simulink model "assignment1"  (R2017b)
settings: Solver=VariableStepAuto  StartTime=0.0  StopTime=10.0  RelTol=1e-3
libraries: hdlsllib x8
settings Model: Creator=Raymond  LastModifiedBy=Raymond

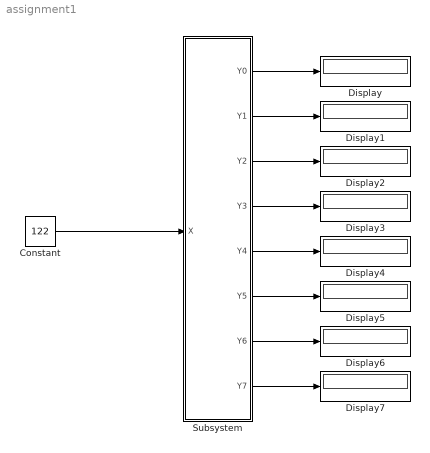
== system assignment1 ==
  Constant : Constant  Value=122  OutDataTypeStr=int8  SampleTime=-1
  Display{,1..7} (8 alike) : Display
  Subsystem : Subsystem
  wires:
  Subsystem/1(Y0) -> Display/1
  Subsystem/2(Y1) -> Display1/1
  Subsystem/3(Y2) -> Display2/1
  Subsystem/4(Y3) -> Display3/1
  Subsystem/5(Y4) -> Display4/1
  Subsystem/6(Y5) -> Display5/1
  Subsystem/7(Y6) -> Display6/1
  Subsystem/8(Y7) -> Display7/1
  Constant/1 -> Subsystem/1(X)

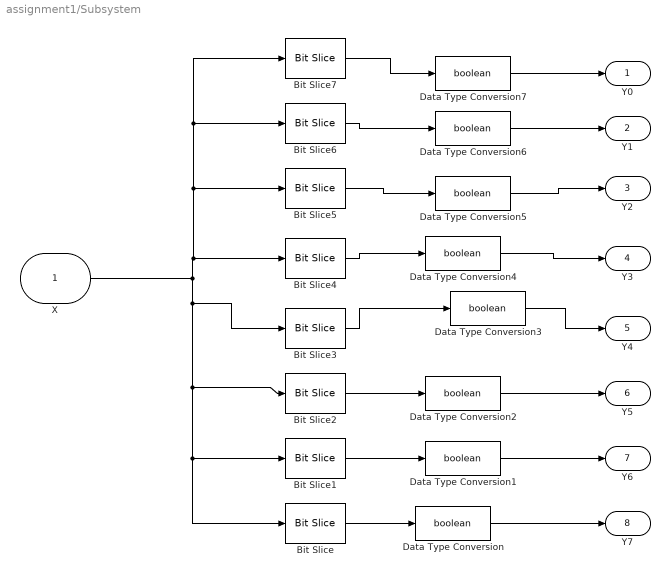
== system assignment1/Subsystem ==
  X : Inport  OutDataTypeStr=int8  SampleTime=1
  Bit Slice : hdlsllib/Logic and Bit Operations/Bit Slice  lidx=7  ridx=7
  Bit Slice1 : hdlsllib/Logic and Bit Operations/Bit Slice  lidx=6  ridx=6
  Bit Slice2 : hdlsllib/Logic and Bit Operations/Bit Slice  lidx=5  ridx=5
  Bit Slice3 : hdlsllib/Logic and Bit Operations/Bit Slice  lidx=4  ridx=4
  Bit Slice4 : hdlsllib/Logic and Bit Operations/Bit Slice  lidx=3  ridx=3
  Bit Slice5 : hdlsllib/Logic and Bit Operations/Bit Slice  lidx=2  ridx=2
  Bit Slice6 : hdlsllib/Logic and Bit Operations/Bit Slice  lidx=1  ridx=1
  Bit Slice7 : hdlsllib/Logic and Bit Operations/Bit Slice  lidx=0  ridx=0
  Data Type Conversion{,1..7} (8 alike) : DataTypeConversion  OutDataTypeStr=boolean
  Y0 : Outport
  Y1 : Outport  Port=2
  Y2 : Outport  Port=3
  Y3 : Outport  Port=4
  Y4 : Outport  Port=5
  Y5 : Outport  Port=6
  Y6 : Outport  Port=7
  Y7 : Outport  Port=8
  wires:
  Data Type Conversion/1 -> Y7/1
  Data Type Conversion1/1 -> Y6/1
  Data Type Conversion6/1 -> Y1/1
  Bit Slice5/1 -> Data Type Conversion5/1
  Data Type Conversion5/1 -> Y2/1
  Data Type Conversion7/1 -> Y0/1
  X/1 -> Bit Slice/1, Bit Slice1/1, Bit Slice2/1, Bit Slice3/1, Bit Slice4/1, Bit Slice5/1, Bit Slice7/1, Bit Slice6/1
  Data Type Conversion3/1 -> Y4/1
  Data Type Conversion4/1 -> Y3/1
  Bit Slice2/1 -> Data Type Conversion2/1
  Bit Slice1/1 -> Data Type Conversion1/1
  Bit Slice/1 -> Data Type Conversion/1
  Data Type Conversion2/1 -> Y5/1
  Bit Slice7/1 -> Data Type Conversion7/1
  Bit Slice6/1 -> Data Type Conversion6/1
  Bit Slice4/1 -> Data Type Conversion4/1
  Bit Slice3/1 -> Data Type Conversion3/1
